simulink model "pulse_oximeter_simulink"  (R2015a)
settings: Solver=ode45  StartTime=0.0  StopTime=10.0  RelTol=1e-3
libraries: simulink x2
settings Model: Creator=Razi Jaam  LastModifiedBy=Razi Jaam

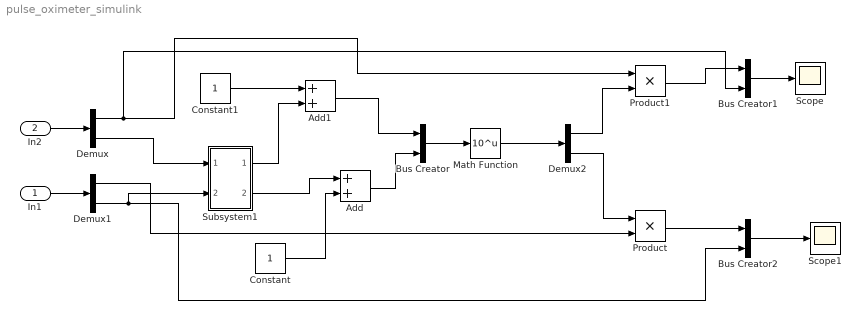
== system pulse_oximeter_simulink ==
  In1 : Inport
  In2 : Inport  Port=2
  Add : Sum
  Add1 : Sum
  Bus Creator : BusCreator  Inputs=2
  Bus Creator1 : BusCreator  Inputs=2
  Bus Creator2 : BusCreator  Inputs=2
  Constant : Constant
  Constant1 : Constant
  Demux : Demux  Outputs=2
  Demux1 : Demux  Outputs=2
  Demux2 : Demux  Outputs=2
  Math Function : Math  Operator=10^u  SaturateOnIntegerOverflow=on
  Product : Product
  Product1 : Product
  Scope : Scope
  Scope1 : Scope
  Subsystem1 : Subsystem
  wires:
  In2/1 -> Demux/1
  Demux/2 -> Subsystem1/1(In1)
  Subsystem1/1(Out1) -> Add1/2
  Constant1/1 -> Add1/1
  Subsystem1/2(Out2) -> Add/1
  Constant/1 -> Add/2
  Add/1 -> Bus Creator/2
  Add1/1 -> Bus Creator/1
  In1/1 -> Demux1/1
  Bus Creator/1 -> Math Function/1
  Math Function/1 -> Demux2/1
  Demux2/1 -> Product1/2
  Demux2/2 -> Product/1
  Demux/1 -> Bus Creator1/2, Product1/1
  Demux1/1 -> Product/2
  Product1/1 -> Bus Creator1/1
  Product/1 -> Bus Creator2/1
  Demux1/2 -> Subsystem1/2(In2), Bus Creator2/2
  Bus Creator1/1 -> Scope/1
  Bus Creator2/1 -> Scope1/1

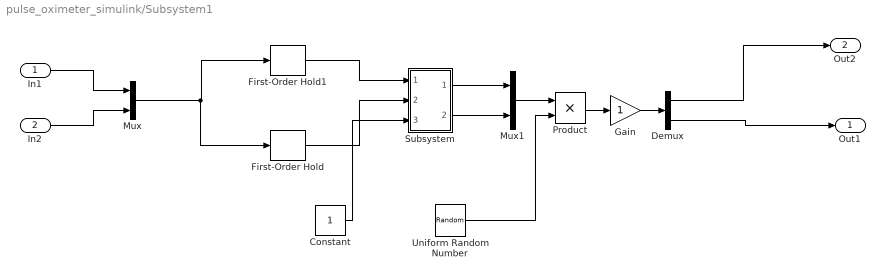
== system pulse_oximeter_simulink/Subsystem1 ==
  In1 : Inport
  In2 : Inport  Port=2
  Constant : Constant
  Demux : Demux  Outputs=2
  First-Order Hold : simulink/Discrete/First-Order Hold  DisableCoverage=on  Ts=1
  First-Order Hold1 : simulink/Discrete/First-Order Hold  DisableCoverage=on  Ts=1
  Gain : Gain
  Mux : Mux  Inputs=2
  Mux1 : Mux  Inputs=2
  Product : Product
  Subsystem : Subsystem
  Uniform Random Number : UniformRandomNumber  SampleTime=0.1
  Out1 : Outport
  Out2 : Outport  Port=2
  wires:
  Uniform Random Number/1 -> Product/2
  Gain/1 -> Demux/1
  Demux/2 -> Out1/1
  Subsystem/1(Out1) -> Mux1/1
  Mux1/1 -> Product/1
  Constant/1 -> Subsystem/3(In3)
  Product/1 -> Gain/1
  Subsystem/2(Out2) -> Mux1/2
  In2/1 -> Mux/2
  First-Order Hold/1 -> Subsystem/2(In2)
  First-Order Hold1/1 -> Subsystem/1(In1)
  Demux/1 -> Out2/1
  Mux/1 -> First-Order Hold/1, First-Order Hold1/1
  In1/1 -> Mux/1

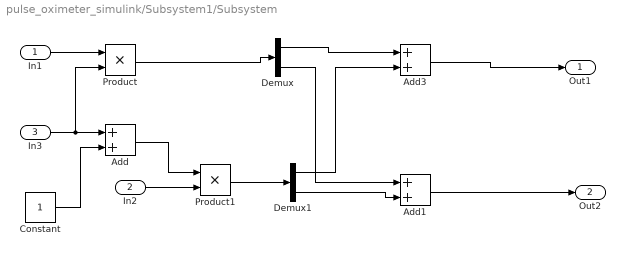
== system pulse_oximeter_simulink/Subsystem1/Subsystem ==
  In1 : Inport
  In2 : Inport  Port=2
  In3 : Inport  Port=3
  Add : Sum
  Add1 : Sum
  Add3 : Sum
  Constant : Constant
  Demux : Demux  Outputs=2
  Demux1 : Demux  Outputs=2
  Product : Product
  Product1 : Product
  Out1 : Outport
  Out2 : Outport  Port=2
  wires:
  Demux1/2 -> Add1/2
  Add/1 -> Product1/1
  Product1/1 -> Demux1/1
  Demux1/1 -> Add3/2
  Add1/1 -> Out2/1
  Demux/2 -> Add1/1
  In3/1 -> Product/2, Add/1
  In1/1 -> Product/1
  Add3/1 -> Out1/1
  In2/1 -> Product1/2
  Constant/1 -> Add/2
  Product/1 -> Demux/1
  Demux/1 -> Add3/1
